simulink model "uz_6ph_ParameterID"  (R2022b)
settings: Solver=FixedStepDiscrete  StartTime=0.0  StopTime=160  FixedStep=0.000005  RelTol=1e-3  EnableMultiTasking=on
model workspace (MATLAB code in the model file):
  | cmdLim = Simulink.Parameter;
  | cmdLim.Value = 15;
  | cmdLim.Description = 'Limit for controlling the maximum surface command angle.';
  | cmdLim.Min = 0;
  | cmdLim.Max = 90;
  | cmdLim.DocUnits = 'deg';
  | 
  | dispGain = Simulink.Parameter;
  | dispGain.Value = 0.75;
  | dispGain.Description = 'Gain applied to the displacement error.';
  | dispGain.Min = 0;
  | dispGain.Max = [];
  | dispGain.DocUnits = 'deg/sec/deg';
  | 
  | dispLim = Simulink.Parameter;
  | dispLim.Value = 30;
  | dispLim.Description = 'Limit for controlling the maximum commanded angle.';
  | dispLim.Min = 0;
  | dispLim.Max = 180;
  | dispLim.DocUnits = 'deg';
  | 
  | intGain = Simulink.Parameter;
  | intGain.Value = 0.5;
  | intGain.Description = 'Gain applied to the integral error.';
  | intGain.Min = 0;
  | intGain.Max = [];
  | intGain.DocUnits = 'deg/sec/deg/sec';
  | 
  | intLim = Simulink.Parameter;
  | intLim.Value = 5;
  | intLim.Description = 'Limit for controlling the maximum commanded angle.';
  | intLim.Min = 0;
  | intLim.Max = 90;
  | intLim.DocUnits = 'deg';
  | 
  | rateGain = Simulink.Parameter;
  | rateGain.Value = 2;
  | rateGain.Description = 'Gain applied to the rate error.';
  | rateGain.Min = 0;
  | rateGain.Max = [];
  | rateGain.DocUnits = 'deg/deg/sec';
  | 
  | rateLim = Simulink.Parameter;
  | rateLim.Value = 6;
  | rateLim.Description = 'Limit for controlling the maximum commanded angle.';
  | rateLim.Min = 0;
  | rateLim.Max = 180;
  | rateLim.DocUnits = 'deg/sec';
  | 
  | hdgGain = Simulink.Parameter;
  | hdgGain.Value = 0.015;
values from neighbouring files (symbols this model uses):
  d_f_states = 20000    [Parameter_Init_Buehler_201.m]
settings Model: RequirementInfo={} %GIDa_fe9045fd_0412_4b6e_8206_617cc20e6fde  FPTRunName=Active  Creator=ts  LastModifiedBy=valen
settings SolverCC: AlgebraicLoopSolver=TrustRegion  PositivePriorityOrder=on  AutoInsertRateTranBlk=on
settings DataIOCC: SaveOutput=off  SignalLogging=off  DSMLogging=off  SaveTime=off
settings OptimizationCC: DefaultParameterBehavior=Inlined  UseDivisionForNetSlopeComputation=on  GainParamInheritBuiltInType=on  UseFloatMulNetSlope=on  DefaultUnderspecifiedDataType=single  UseSpecifiedMinMax=on  InlineInvariantSignals=on  PassReuseOutputArgsAs=Individual arguments  NoFixptDivByZeroProtection=on  EfficientFloat2IntCast=on  LifeSpan=1  MaxStackSize=64  OptimizeBlockOrder=speed  DifferentSizesBufferReuse=on  EfficientTunableParamExpr=on
settings DebuggingCC: UnconnectedInputMsg=warning  UnconnectedOutputMsg=warning  UnconnectedLineMsg=warning  BusObjectLabelMismatch=error  AllowSymbolicDim=off  SFUnexpectedBacktrackingDiag=warning  SFNoUnconditionalDefaultTransitionDiag=warning  SFExecutionAtInitializationDiag=none  SFMachineParentedDataDiag=warning  ArithmeticOperatorsInVariantConditions=warning
settings HardwareCC: ProdBitPerPointer=32  ProdBitPerSizeT=32  ProdBitPerPtrDiffT=32  ProdLargestAtomicInteger=Long  ProdLargestAtomicFloat=Double  ProdWordSize=32  ProdLongLongMode=on  ProdHWDeviceType=ARM Compatible->ARM Cortex-R  HardwareBoardFeatureSet=SoCBlockset
settings ModelReferenceCC: EnableRefExpFcnMdlSchedulingChecks=on
settings SFSimCC: SimGenImportedTypeDefs=on  MATLABDynamicMemAlloc=off
settings RTWCC: Description=Embedded Coder  SystemTargetFile=ert.tlc  GenCodeOnly=on  TemplateMakefile=ert_default_tmf  GenerateReport=on  BuildConfiguration=Faster Runs  IncludeHyperlinkInReport=on  GenerateTraceInfo=on  GenerateTraceReport=on  GenerateTraceReportSl=on  GenerateTraceReportSf=on  GenerateTraceReportEml=on  GenerateCodeMetricsReport=on  CheckMdlBeforeBuild=Warning  DLArmComputeVersion=19.05
settings CodeAppCC: ForceParamTrailComments=on  IgnoreCustomStorageClasses=off  OperatorAnnotations=on  SimulinkDataObjDesc=on  SFDataObjDesc=on  MATLABFcnDesc=on  CustomSymbolStrGlobalVar=rt$M$R$N  CustomSymbolStrType=$N$M$R_t  CustomSymbolStrFcn=$N$M$F  CustomSymbolStrMacro=$N$M  InsertBlockDesc=on  StateflowObjectComments=on  MATLABSourceComments=on  EnableCustomComments=on  ReqsInCode=on
settings ERTTargetCC: TargetLangStandard=C99 (ISO)  CodeReplacementLibrary=GNU C99 extensions  UtilityFuncGeneration=Shared location  MultiwordLength=2048  IncludeMdlTerminateFcn=off  CombineSignalStateStructs=on  SuppressErrorStatus=on  IncludeFileDelimiter=UseQuote  SupportAbsoluteTime=off  CodeInterfacePackaging=Reusable function  SupportNonFinite=off  RemoveResetFunc=off  InlinedParameterPlacement=NonHierarchical  MultiInstanceErrorCode=Warning  RootIOFormat=Part of model data structure  ERTCustomFileTemplate=example_file_process.tlc  GlobalDataDefinition=InSeparateSourceFile  DataDefinitionFile=hallohaloo.c  GlobalDataReference=InSeparateHeaderFile  ERTFilePackagingFormat=CompactWithDataFile  DataReferenceFile=uz_ParameterID_data.h  SuppressUnreachableDefaultCases=off  EnableSignedRightShifts=off
settings ConfigComp: CovScope=ReferencedModels  CovSaveName=covdata_rollAP  CovMetricSettings=dcmtrwe  CovHTMLOptions=-sRT=1 -aTS=1 -bRG=1 -bTC=1 -hTR=1 -nFC=0 -scm=1 -bcm=1 -xEv=0  CovSaveCumulativeToWorkspaceVar=on  CovSaveSingleToWorkspaceVar=on  CovCumulativeVarName=covCumulativeData_rollAP  CovReportOnPause=off  CovExternalEMLEnable=off  CovSFcnEnable=off

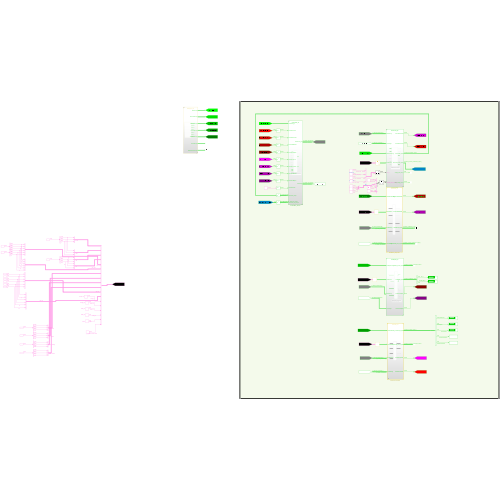
[thumbnail: Simulink's stored preview of the top-level diagram]
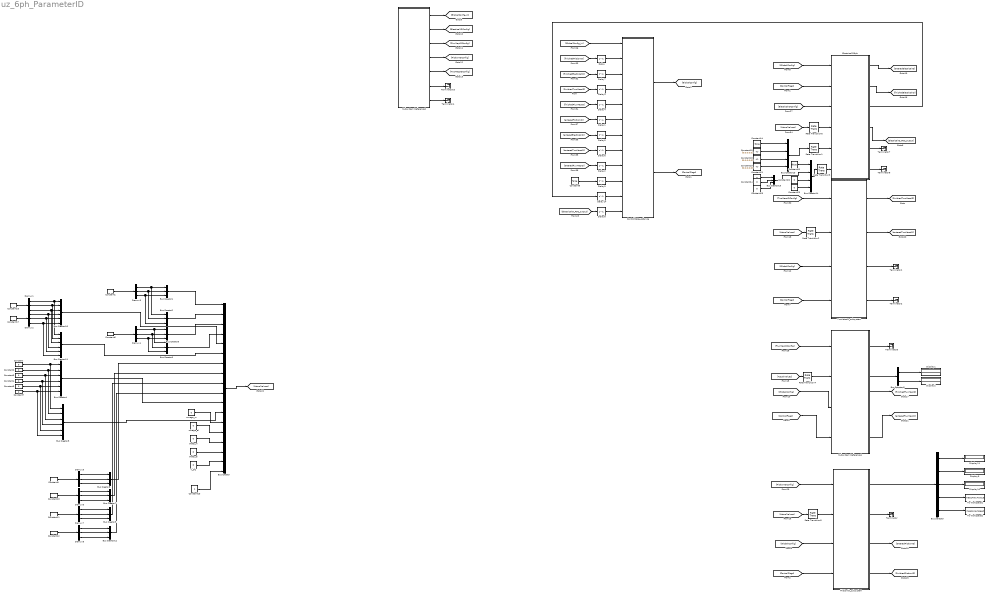
== system uz_6ph_ParameterID ==
  Bus Creator : BusCreator  Inputs=18  OutDataTypeStr=Bus: uz_ParaID_ActualValues_t
  Bus Creator1 : BusCreator  Inputs=3  OutDataTypeStr=Bus: uz_3ph_abc_t
  Bus Creator10 : BusCreator  Inputs=6  OutDataTypeStr=Bus: uz_6ph_abc_t
  Bus Creator11 : BusCreator  Inputs=6  OutDataTypeStr=Bus: uz_6ph_abc_t
  Bus Creator{5..9,12,15} (7 alike) : BusCreator  Inputs=3  OutDataTypeStr=Bus: uz_3ph_dq_t
  Bus Creator13 : BusCreator  Inputs=4  OutDataTypeStr=Bus: uz_ParaID_ElectricalID_fft_in_t
  Bus Creator14 : BusCreator  Inputs=4  OutDataTypeStr=Bus: uz_ParaID_ElectricalID_offset_estimation_t
  Bus Creator2 : BusCreator  Inputs=3  OutDataTypeStr=Bus: uz_3ph_abc_t
  Bus Creator3 : BusCreator  Inputs=6  OutDataTypeStr=Bus: uz_6ph_dq_t
  Bus Creator4 : BusCreator  Inputs=6  OutDataTypeStr=Bus: uz_6ph_dq_t
  Bus Selector : BusSelector  OutputSignals=BrkTorque,CoulTorque,ViscoTorque,measArrayTorque,measArraySpeed
  Bus Selector5 : BusSelector  OutputSignals=R_s,WindingTemp
  Constant{,2..5,7,21..25} (11 alike) : Constant  Value=0  OutDataTypeStr=single
  Constant{1,6,9..12,16..17} (8 alike) : Constant  Value=[0;0;0]  OutDataTypeStr=single
  Constant13 : Constant  OutDataTypeStr=single
  Constant14 : Constant  Value=false  OutDataTypeStr=boolean
  Constant15 : Constant  Value=[0,0,0,0,0]  OutDataTypeStr=single
  Constant18 : Constant  Value=[0,0,0,0,0]  OutDataTypeStr=single
  Constant19 : Constant  Value=[0,0,0,0,0]  OutDataTypeStr=single
  Constant20 : Constant  Value=false  OutDataTypeStr=boolean
  Constant8 : Constant  Value=false  OutDataTypeStr=boolean
  ControlState_refernce : Subsystem  ReferencedSubsystem=ControlState_ref
  Delay{,1..9,14} (11 alike) : Delay  DelayLength=1  InitialCondition=0
  Demux{1..8} (8 alike) : Demux  Outputs=3
  Display{1..2,9..11} (5 alike) : Display
  ElectricalID6ph : Subsystem  ReferencedSubsystem=ElectricalID_6ph
  FrictionID_subsystem : ModelReference  ModelNameDialog=FrictionID_ref.slx  SimulationMode=Normal  ModelReferenceVersion=5.45
      settings: PortSchema="{\"entries\":[{\"content\":{\"sides\":[{\"content\":{\"connectorIds\":[\"In1\",\"In2\",\"In3\",\"In4\"]},\"type\":\"ConnectorPlacement.EquallySpacedRectSide\",\"uuid\":\"9228c284-4dde-45fc-9186-6f631f78e5bf\"},{\"content\":{\"connectorIds\":[\"Out4\",\"Out3\",\"Out2\",\"Out1\"],\"side\":\"RIGHT\"},\"type\":\"ConnectorPlacement.EquallySpacedRectSide\",\"uuid\":\"71961043-480b-43aa-8cdd-23d9057d5ad4\"},{\"content\":{\"connectorIds\":[],\"side\":\"TOP\"},\"type\":\"ConnectorPlacement.EquallySpacedRectSide\",\"uuid\":\"f6f3bc9d-566f-4498-bf43-24e8b901b7a7\"}]},\"type\":\"ConnectorPlacement.EquallySpacedConnector\",\"uuid\":\"83d2d7c4-30d1-4ed4-b102-cbae6a0e9817\"}],\"packageUris\":[\"http://schema.mathworks.com/mf0/Connector/R2020b\"],\"version\":\"1.0\"}"
  Rate Transition{1..6} (6 alike) : RateTransition  OutPortSampleTime=1/d_f_states
  Subsystem Reference1 : Subsystem  ReferencedSubsystem=FluxMapID_6ph
  Subsystem Reference2 : Subsystem  ReferencedSubsystem=model_bus_init
  Terminator{,1..4,7..8,10} (8 alike) : Terminator
  To Workspace1 : ToWorkspace  VariableName=measArrayTorque  SampleTime=-1
      settings: MaxDataPoints=1
  To Workspace2 : ToWorkspace  VariableName=measArraySpeed  SampleTime=-1
      settings: MaxDataPoints=1
  TwoMassID_subsystem : ModelReference  ModelNameDialog=TwoMassID_ref.slx  SimulationMode=Normal  ModelReferenceVersion=5.45
      settings: PortSchema="{\"entries\":[{\"content\":{\"sides\":[{\"content\":{\"connectorIds\":[\"In1\",\"In2\",\"In3\",\"In4\"]},\"type\":\"ConnectorPlacement.EquallySpacedRectSide\",\"uuid\":\"b3f846b4-67b8-414d-80f8-2cdf230e8050\"},{\"content\":{\"connectorIds\":[\"Out1\",\"Out2\",\"Out4\",\"Out3\"],\"side\":\"RIGHT\"},\"type\":\"ConnectorPlacement.EquallySpacedRectSide\",\"uuid\":\"f153ecc1-7a63-46b5-bb71-72b88e4117b7\"},{\"content\":{\"connectorIds\":[],\"side\":\"TOP\"},\"type\":\"ConnectorPlacement.EquallySpacedRectSide\",\"uuid\":\"7aaf7a4c-17fe-4dd1-8ce1-675b09504e17\"}]},\"type\":\"ConnectorPlacement.EquallySpacedConnector\",\"uuid\":\"e21480e7-4483-4a1e-b62d-5327482c3f88\"}],\"packageUris\":[\"http://schema.mathworks.com/mf0/Connector/R2020b\"],\"version\":\"1.0\"}"
  V_DC : Constant  Value=0  OutDataTypeStr=single
  omega_el : Constant  Value=0  OutDataTypeStr=single
  omega_m : Constant  Value=0  OutDataTypeStr=single
  theta_el : Constant  Value=0  OutDataTypeStr=single
  theta_m : Constant  Value=0  OutDataTypeStr=single
  wires:
  Bus Selector/3 -> Display10/1  "<ViscoTorque>"
  Subsystem Reference2/5 -> [TwoMassIDConfig]
  [finishedFrictionID] -> Delay/1
  Delay/1 -> ControlState_refernce/2
  Subsystem Reference2/1 -> [GlobalConfig_in]
  Delay14/1 -> ControlState_refernce/11
  Delay2/1 -> ControlState_refernce/9
  Delay5/1 -> ControlState_refernce/7
  Delay6/1 -> ControlState_refernce/8
  [enteredElectricalID] -> Delay5/1
  [enteredFrictionID] -> Delay1/1
  [finishedFluxMapID] -> Delay4/1
  [finishedTwoMassID] -> Delay3/1
  Subsystem Reference2/2 -> [ElectricalIDConfig]
  Subsystem Reference2/4 -> [FrictionIDConfig]
  Bus Selector/1 -> Display11/1  "<BrkTorque>"
  Delay1/1 -> ControlState_refernce/6
  [ElectricalID_FOC_output] -> Delay8/1
  Delay7/1 -> ControlState_refernce/3
  [ActualValues] -> Rate Transition6/1
  Delay8/1 -> ControlState_refernce/12
  ControlState_refernce/1 -> [GlobalConfig]
  [ActualValues] -> Rate Transition2/1
  Subsystem Reference2/6 -> Terminator10/1
  Bus Selector5/1 -> Display1/1  "<R_s>"
  [GlobalConfig_in] -> ControlState_refernce/1
  Delay3/1 -> ControlState_refernce/4
  Subsystem Reference2/3 -> [FluxMapIDConfig]
  Bus Selector/2 -> Display9/1  "<CoulTorque>"
  ControlState_refernce/2 -> [ControlFlags]
  [ActualValues] -> Rate Transition4/1
  Delay4/1 -> ControlState_refernce/5
  [finishedElectricalID] -> Delay7/1
  [ActualValues] -> Rate Transition5/1
  [enteredFluxMapID] -> Delay2/1
  [enteredTwoMassID] -> Delay6/1
  Bus Selector5/2 -> Display2/1  "<WindingTemp>"
  omega_el/1 -> Bus Creator/14  "omega_el"
  Bus Creator/1 -> [ActualValues]
  omega_m/1 -> Bus Creator/13  "omega_m"
  theta_m/1 -> Bus Creator/15  "theta_m"
  V_DC/1 -> Bus Creator/17  "V_DC"
  theta_el/1 -> Bus Creator/16  "theta_el"
  Subsystem Reference2/7 -> Terminator4/1
  Delay9/1 -> ControlState_refernce/10
  Constant8/1 -> Delay9/1
  Bus Selector/4 -> To Workspace1/1  "<measArrayTorque>"
  Bus Selector/5 -> To Workspace2/1  "<measArraySpeed>"
  [FrictionIDConfig] -> FrictionID_subsystem/1
  [GlobalConfig] -> FrictionID_subsystem/3
  [ControlFlags] -> FrictionID_subsystem/4
  FrictionID_subsystem/4 -> Bus Selector/1
  FrictionID_subsystem/3 -> Terminator/1
  FrictionID_subsystem/2 -> [enteredFrictionID]
  FrictionID_subsystem/1 -> [finishedFrictionID]
  [FluxMapIDConfig] -> Subsystem Reference1/1
  [GlobalConfig] -> Subsystem Reference1/3
  [ControlFlags] -> Subsystem Reference1/4
  Subsystem Reference1/1 -> Terminator3/1
  Subsystem Reference1/2 -> Bus Selector5/1
  Subsystem Reference1/3 -> [finishedFluxMapID]
  Subsystem Reference1/4 -> [enteredFluxMapID]
  ElectricalID6ph/3 -> Delay14/1
  [GlobalConfig] -> ElectricalID6ph/1
  [ControlFlags] -> ElectricalID6ph/2
  [ElectricalIDConfig] -> ElectricalID6ph/3
  Rate Transition6/1 -> ElectricalID6ph/4
  ElectricalID6ph/1 -> [enteredElectricalID]
  ElectricalID6ph/2 -> [finishedElectricalID]
  ElectricalID6ph/4 -> [ElectricalID_FOC_output]
  [TwoMassIDConfig] -> TwoMassID_subsystem/1
  [GlobalConfig] -> TwoMassID_subsystem/3
  [ControlFlags] -> TwoMassID_subsystem/4
  TwoMassID_subsystem/1 -> [finishedTwoMassID]
  TwoMassID_subsystem/2 -> [enteredTwoMassID]
  Rate Transition2/1 -> TwoMassID_subsystem/2
  Rate Transition4/1 -> Subsystem Reference1/2
  Rate Transition5/1 -> FrictionID_subsystem/2
  Demux1/3 -> Bus Creator11/3, Bus Creator10/3  "c1"
  Demux1/2 -> Bus Creator11/2, Bus Creator10/2  "b1"
  Constant17/1 -> Demux2/1
  Constant16/1 -> Demux1/1
  Demux2/1 -> Bus Creator11/4, Bus Creator10/4  "a2"
  Demux2/3 -> Bus Creator11/6, Bus Creator10/6  "c2"
  Demux1/1 -> Bus Creator11/1, Bus Creator10/1  "a1"
  Demux2/2 -> Bus Creator11/5, Bus Creator10/5  "b2"
  Bus Creator11/1 -> Bus Creator/6  "i_abc_6ph"
  Constant2/1 -> Bus Creator3/2, Bus Creator4/2  "q"
  Constant3/1 -> Bus Creator3/3, Bus Creator4/3  "x"
  Constant/1 -> Bus Creator3/1, Bus Creator4/1  "d"
  Bus Creator4/1 -> Bus Creator/11  "i_dq_6ph"
  Constant4/1 -> Bus Creator3/4, Bus Creator4/4  "y"
  Bus Creator3/1 -> Bus Creator/12  "v_dq_6ph"
  Constant5/1 -> Bus Creator3/5, Bus Creator4/5  "z1"
  Constant7/1 -> Bus Creator3/6, Bus Creator4/6  "z2"
  Demux3/3 -> Bus Creator2/3, Bus Creator1/3  "c"
  Demux3/1 -> Bus Creator2/1, Bus Creator1/1  "a"
  Demux3/2 -> Bus Creator2/2, Bus Creator1/2  "b"
  Constant1/1 -> Demux3/1
  Bus Creator1/1 -> Bus Creator/1  "V_abc"
  Bus Creator2/1 -> Bus Creator/2  "I_abc"
  Bus Creator5/1 -> Bus Creator/3  "i_dq"
  Constant6/1 -> Demux4/1
  Demux4/3 -> Bus Creator6/3, Bus Creator5/3  "zero"
  Demux4/1 -> Bus Creator6/1, Bus Creator5/1  "d"
  Demux4/2 -> Bus Creator6/2, Bus Creator5/2  "q"
  Bus Creator6/1 -> Bus Creator/4  "v_dq"
  ElectricalID6ph/5 -> Terminator7/1
  ElectricalID6ph/6 -> Terminator8/1
  Demux5/2 -> Bus Creator8/2  "q"
  Demux5/1 -> Bus Creator8/1  "d"
  Demux5/3 -> Bus Creator8/3  "zero"
  Constant9/1 -> Demux5/1
  Bus Creator8/1 -> Bus Creator/7  "v_xy_rotating"
  Bus Creator10/1 -> Bus Creator/5  "v_abc_6ph"
  Constant10/1 -> Demux6/1
  Demux6/3 -> Bus Creator7/3  "zero"
  Demux6/1 -> Bus Creator7/1  "d"
  Demux6/2 -> Bus Creator7/2  "q"
  Demux7/2 -> Bus Creator9/2  "q"
  Demux7/1 -> Bus Creator9/1  "d"
  Demux7/3 -> Bus Creator9/3  "zero"
  Constant11/1 -> Demux7/1
  Constant12/1 -> Demux8/1
  Demux8/3 -> Bus Creator12/3  "zero"
  Demux8/1 -> Bus Creator12/1  "d"
  Demux8/2 -> Bus Creator12/2  "q"
  Bus Creator7/1 -> Bus Creator/8  "i_xy_rotating"
  Bus Creator9/1 -> Bus Creator/9  "v_zero_rotating"
  Bus Creator12/1 -> Bus Creator/10  "i_zero_rotating"
  Constant13/1 -> Bus Creator/18  "average_winding_temp"
  TwoMassID_subsystem/4 -> Terminator1/1
  TwoMassID_subsystem/3 -> Terminator2/1
  Bus Creator13/1 -> Rate Transition1/1
  Constant14/1 -> Bus Creator13/1  "finished_flag"
  Constant15/1 -> Bus Creator13/2  "psi_pm_frequency"
  Constant19/1 -> Bus Creator13/4  "psi_pm_angle"
  Constant18/1 -> Bus Creator13/3  "psi_pm_amplitude"
  Constant22/1 -> Bus Creator14/3  "progress"
  Constant23/1 -> Bus Creator14/4  "offset_angle_rad"
  Bus Creator15/1 -> Bus Creator14/2  "i_dq_ref"
  Constant20/1 -> Bus Creator14/1  "finished_flag"
  Constant21/1 -> Bus Creator15/1  "d"
  Constant24/1 -> Bus Creator15/2  "q"
  Constant25/1 -> Bus Creator15/3  "zero"
  Rate Transition1/1 -> ElectricalID6ph/5
  Rate Transition3/1 -> ElectricalID6ph/6
  Bus Creator14/1 -> Rate Transition3/1
